simulink model "IPMSM_dq_Fault_R2020b_M"  (R2020b)
settings: Solver=VariableStepAuto  StartTime=0.0  StopTime=0.4  RelTol=1e-3
InitFcn:
  | clc
  | p=2;
  | R=3.45;
  | Ld=9.5e-3;
  | Lq=12e-3;
  | flux=0.55;
  | B=0;
  | J=0.0052;
  | 
  | L=(Ld+Lq)/2;
  | M=0.5e-3;
  | 
  | Rf=0.5;
  | 
  | TL=1e-6;
  | 
  | Ts=1e-6;
libraries: powerlib x6, powerlib_extras x3, simulink x1
settings Model: SimulationMode=accelerator  Creator=acer  LastModifiedBy=Beyond
settings DataIOCC: ReturnWorkspaceOutputs=off
settings DebuggingCC: ArithmeticOperatorsInVariantConditions=warning
settings SFSimCC: CustomCodeUndefinedFunction=UseInterfaceOnly
settings CodeAppCC: StateflowObjectComments=on

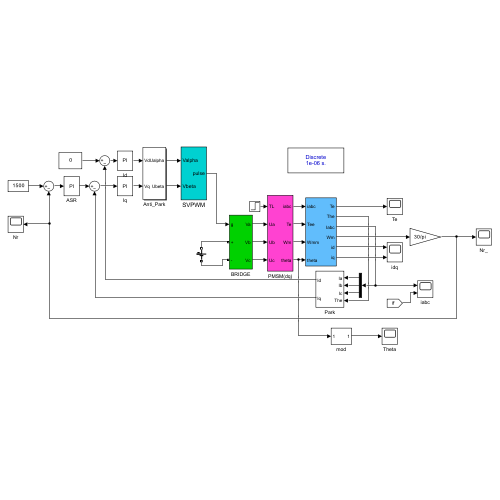
[thumbnail: Simulink's stored preview of the top-level diagram]
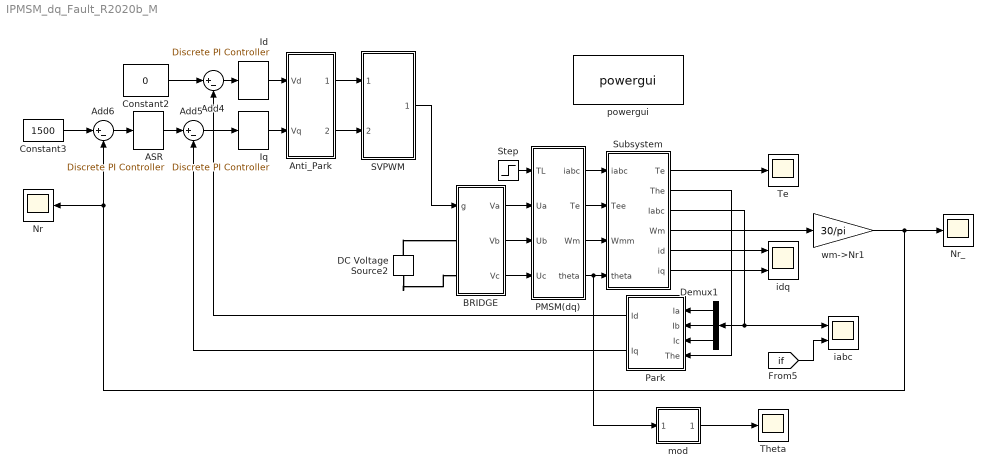
== system IPMSM_dq_Fault_R2020b_M ==
  ASR : powerlib_extras/Discrete  Control Blocks/Discrete PI Controller  Kp=0.15  Ki=10  Par_Limits=[30 -30]  Init=0  Ts=Ts
  Add4 : Sum  Inputs=|+-
  Add5 : Sum  Inputs=|+-
  Add6 : Sum  Inputs=|+-
  Anti_Park : Subsystem
  BRIDGE : Subsystem
  Constant2 : Constant  Value=0
  Constant3 : Constant  Value=1500
  DC Voltage Source2 : powerlib/Electrical Sources/DC Voltage Source  Amplitude=500  Measurements=None
  Demux1 : Demux  Outputs=3
  Id : powerlib_extras/Discrete  Control Blocks/Discrete PI Controller  Kp=Ld*5000  Ki=R*5000  Par_Limits=[500*0.9*sqrt(1/3) -500*0.9*sqrt(1/3)]  Init=0  Ts=Ts
  Iq : powerlib_extras/Discrete  Control Blocks/Discrete PI Controller  Kp=Lq*5000  Ki=R*5000  Par_Limits=[500*0.9*sqrt(1/3) -500*0.9*sqrt(1/3)]  Init=0  Ts=Ts
  Nr : Scope
  Nr_ : Scope
  PMSM(dq) : Subsystem
  Park : Subsystem
  SVPWM : Subsystem
  Step : Step  Time=0.1  Before=2  After=20  SampleTime=0
  Subsystem : Subsystem
  Te : Scope
  Theta : Scope
  iabc : Scope  NumInputPorts=2
  idq : Scope  NumInputPorts=2
  mod : Subsystem
  powergui : powerlib/powergui  SimulationMode=Discrete  SampleTime=1e-6  frequency=60  Iterations=50  frequencyindice=0  Pbase=100e6  ErrMax=1e-4  UnitsV=kV  UnitsW=MW  buscounter=0  FunctionMessages=off  echomessages=off  EnableUseOfTLC=off  CurrentSourceSwitches=off  DisableSnubberDevices=off  DisableRonSwitches=off  DisableVfSwitches=off  DisplayEquations=off  AutomaticDiscreteSolvers=off  SolverType=Tustin/Backward Euler (TBE)  Interpol=off  ExternalGateDelay=off  methode=off  Ts=100  x0status=blocks  SPID=off  SwTol=0  HookPort=off  NonlinearTolerance=1e-4  nMaxIteration=100  ContinueOnMaxIteration=off  RestoreLinks=warning  ResistiveCurrentMeasurement=off  Frange=[0:2:500]  Ylog=off  Xlog=on  ShowGrid=off  save=off  variable=ZData  structure=0  ZoomFFT=off  StartTime=0.0  cycles=1  DisplayStyle=1  fundamental=60  FreqAxis=off  MaxFrequency=1000  frequencyindicesteady=1  RmsSteady=1  display=off
  wm->Nr1 : Gain  Gain=30/pi
  wires:
  Id/1 -> Anti_Park/1(Vd)
  PMSM(dq)/3(Wm) -> Subsystem/3(Wmm)
  PMSM(dq)/2(Te) -> Subsystem/2(Tee)
  Park/1(Id) -> Add4/2
  Demux1/1 -> Park/1(Ia)
  PMSM(dq)/1(iabc) -> Subsystem/1(iabc)
  SVPWM/1(pulse) -> BRIDGE/1(g)
  Step/1 -> PMSM(dq)/1("TL ")
  Add5/1 -> Iq/1
  Anti_Park/2(Ubeta) -> SVPWM/2(Vbeta)
  Subsystem/2(The) -> Park/4(The)
  Subsystem/3(Iabc) -> iabc/1, Demux1/1
  Demux1/2 -> Park/2(Ib)
  Subsystem/6(iq) -> idq/2
  Subsystem/1(Te) -> Te/1
  Iq/1 -> Anti_Park/2(Vq)
  ASR/1 -> Add5/1
  Demux1/3 -> Park/3(Ic)
  Add4/1 -> Id/1
  Add6/1 -> ASR/1
  Subsystem/5(id) -> idq/1
  Anti_Park/1(Ualpha) -> SVPWM/1(Valpha)
  Constant2/1 -> Add4/1
  Constant3/1 -> Add6/1
  Park/2(Iq) -> Add5/2
  BRIDGE/1(Va) -> PMSM(dq)/2(Ua)
  BRIDGE/2(Vb) -> PMSM(dq)/3(Ub)
  BRIDGE/3(Vc) -> PMSM(dq)/4(Uc)
  wm->Nr1/1 -> Nr_/1, Nr/1, Add6/2
  mod/1(Out1) -> Theta/1
  PMSM(dq)/4(theta) -> mod/1(In1), Subsystem/4(theta)
  Subsystem/4(Wm) -> wm->Nr1/1
  [if] -> iabc/2
  connections:
  DC Voltage Source2/LConn1 -- BRIDGE/LConn2
  DC Voltage Source2/RConn1 -- BRIDGE/LConn1

== system IPMSM_dq_Fault_R2020b_M/Anti_Park ==
  Vd : Inport
  Vq : Inport  Port=2
  Fcn : Fcn  Expr=cos(u[3])*u[1]-sin(u[3])*u[2]
  Fcn1 : Fcn  Expr=sin(u[3])*u[1]+cos(u[3])*u[2]
  Mux1 : Mux  Inputs=3
  Ualpha : Outport
  Ubeta : Outport  Port=2
  wires:
  Fcn1/1 -> Ubeta/1
  Fcn/1 -> Ualpha/1
  Mux1/1 -> Fcn/1, Fcn1/1
  Vd/1 -> Mux1/1
  Vq/1 -> Mux1/2
  [Thedq] -> Mux1/3

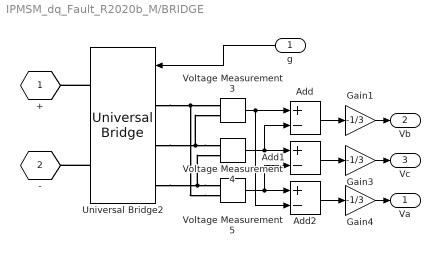
== system IPMSM_dq_Fault_R2020b_M/BRIDGE ==
  g : Inport
  Add : Sum  Inputs=+-
  Add1 : Sum  Inputs=+-
  Add2 : Sum  Inputs=+-
  Gain1 : Gain  Gain=-1/3
  Gain3 : Gain  Gain=-1/3
  Gain4 : Gain  Gain=-1/3
  Universal Bridge2 : powerlib/Power Electronics/Universal Bridge  Arms=3  SnubberResistance=1e5  SnubberCapacitance=inf  Device=IGBT / Diodes  Ron=1e-3  Lon=0  ForwardVoltages="[  0  0  ]"  ForwardVoltage=0  GTOparameters=[ 10e-6 , 20e-6 ]  IGBTparameters=[ 1e-6 , 2e-6 ]  Measurements=None  Measurements_2=None  converterType=Rectifier
  Voltage Measurement3 : powerlib/Measurements/Voltage Measurement  PhasorSimulation=off  OutputType=Complex  PSBequivalent=0
  Voltage Measurement4 : powerlib/Measurements/Voltage Measurement  PhasorSimulation=off  OutputType=Complex  PSBequivalent=0
  Voltage Measurement5 : powerlib/Measurements/Voltage Measurement  PhasorSimulation=off  OutputType=Complex  PSBequivalent=0
  + : PMIOPort  Tag=PMCPort  Side=Left
  - : PMIOPort  Tag=PMCPort  Port=2  Side=Left
  Va : Outport
  Vb : Outport  Port=2
  Vc : Outport  Port=3
  wires:
  g/1 -> Universal Bridge2/1
  Gain1/1 -> Vb/1
  Add2/1 -> Gain4/1
  Gain4/1 -> Va/1
  Voltage Measurement3/1 -> Add/1, Add2/2
  Voltage Measurement4/1 -> Add1/1, Add/2
  Add1/1 -> Gain3/1
  Voltage Measurement5/1 -> Add2/1, Add1/2
  Gain3/1 -> Vc/1
  Add/1 -> Gain1/1
  connections:
  Universal Bridge2/RConn1 -- +/RConn1
  Universal Bridge2/RConn2 -- -/RConn1
  Voltage Measurement5/LConn2 -- Universal Bridge2/LConn1 -- Voltage Measurement3/LConn1
  Voltage Measurement5/LConn1 -- Universal Bridge2/LConn3 -- Voltage Measurement4/LConn2
  Voltage Measurement4/LConn1 -- Universal Bridge2/LConn2 -- Voltage Measurement3/LConn2

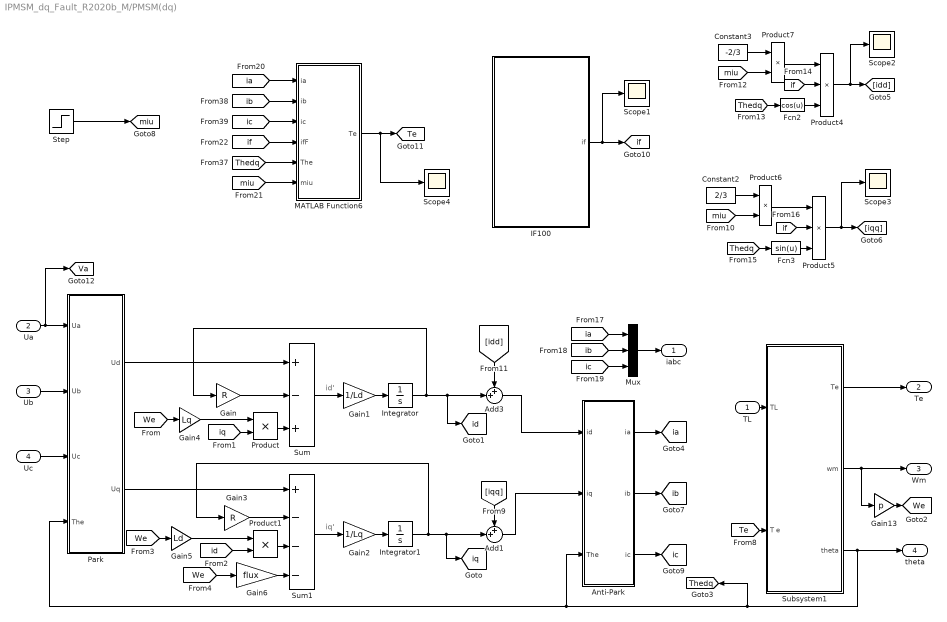
== system IPMSM_dq_Fault_R2020b_M/PMSM(dq) ==
  note: iq'
  note: id'
  "TL " : Inport
  Ua : Inport  Port=2
  Ub : Inport  Port=3
  Uc : Inport  Port=4
  Add1 : Sum  Inputs=++|
  Add3 : Sum  Inputs=++|
  Anti-Park : Subsystem
  Constant2 : Constant  Value=2/3
  Constant3 : Constant  Value=-2/3
  Fcn2 : Fcn  Expr=cos(u)
  Fcn3 : Fcn  Expr=sin(u)
  Gain : Gain  Gain=R
  Gain1 : Gain  Gain=1/Ld
  Gain13 : Gain  Gain=p
  Gain2 : Gain  Gain=1/Lq
  Gain3 : Gain  Gain=R
  Gain4 : Gain  Gain=Lq
  Gain5 : Gain  Gain=Ld
  Gain6 : Gain  Gain=flux
  IF100 : Subsystem
  Integrator : Integrator
  Integrator1 : Integrator
  MATLAB Function6 : MATLAB Function  TreatAsAtomicUnit=on
  Mux : Mux  Inputs=3
  Park : Subsystem
  Product{,1,6..7} (4 alike) : Product
  Product4 : Product  Inputs=3
  Product5 : Product  Inputs=3
  Scope{1..4} (4 alike) : Scope
  Step : Step  Time=0.2  After=0.12  SampleTime=0
  Subsystem1 : Subsystem
  Sum : Sum  Inputs=+-+
  Sum1 : Sum  Inputs=+---
  iabc : Outport
  Te : Outport  Port=2
  Wm : Outport  Port=3
  theta : Outport  Port=4
  tag scope: Te=global, Thedq=global, Va=global, We=global, ia=global, ib=global, ic=global, id=global, if=global, iq=global, miu=global
  wires:
  Ua/1 -> [Va], Park/1(Ua)
  Gain/1 -> Sum/2
  Sum/1 -> Gain1/1
  Subsystem1/1(Te) -> Te/1
  Gain4/1 -> Product/1
  Gain6/1 -> Sum1/4
  [id] -> Product1/2
  Ub/1 -> Park/2(Ub)
  Gain2/1 -> Integrator1/1
  [We] -> Gain6/1
  Subsystem1/3(theta) -> theta/1, [Thedq], Park/4(The), Anti-Park/3(The)
  Product1/1 -> Sum1/3
  [iq] -> Product/2
  Gain5/1 -> Product1/1
  Park/1(Ud) -> Sum/1
  Product/1 -> Sum/3
  Gain3/1 -> Sum1/2
  Gain1/1 -> Integrator/1
  Park/2(Uq) -> Sum1/1
  Subsystem1/2(wm) -> Gain13/1, Wm/1
  Sum1/1 -> Gain2/1
  Gain13/1 -> [We]
  [We] -> Gain4/1
  "TL "/1 -> Subsystem1/1(TL)
  [We] -> Gain5/1
  Uc/1 -> Park/3(Uc)
  Integrator/1 -> [id], Add3/2, Gain/1
  Integrator1/1 -> Gain3/1, [iq], Add1/2
  [idd] -> Add3/1
  [iqq] -> Add1/1
  Add3/1 -> Anti-Park/1(id)
  Add1/1 -> Anti-Park/2(iq)
  Product5/1 -> Scope3/1, [iqq]
  Product7/1 -> Product4/1
  [if] -> Product4/2
  Constant2/1 -> Product6/1
  [Thedq] -> Fcn3/1
  [miu] -> Product7/2
  Product6/1 -> Product5/1
  Fcn2/1 -> Product4/3
  Product4/1 -> Scope2/1, [idd]
  Constant3/1 -> Product7/1
  [Thedq] -> Fcn2/1
  [miu] -> Product6/2
  Fcn3/1 -> Product5/3
  [if] -> Product5/2
  Step/1 -> [miu]
  Anti-Park/1(ia) -> [ia]
  Anti-Park/2(ib) -> [ib]
  Anti-Park/3(ic) -> [ic]
  [Te] -> Subsystem1/2(T e)
  Mux/1 -> iabc/1
  [ia] -> Mux/1
  [ib] -> Mux/2
  [ic] -> Mux/3
  MATLAB Function6/1(Te) -> Scope4/1, [Te]
  [ia] -> MATLAB Function6/1(ia)
  [Thedq] -> MATLAB Function6/5(The)
  [ic] -> MATLAB Function6/3(ic)
  [ib] -> MATLAB Function6/2(ib)
  [if] -> MATLAB Function6/4(ifF)
  [miu] -> MATLAB Function6/6(miu)
  IF100/1(if) -> [if], Scope1/1

== system IPMSM_dq_Fault_R2020b_M/Park ==
  Ia : Inport
  Ib : Inport  Port=2
  Ic : Inport  Port=3
  The : Inport  Port=4
  Mux : Mux
  d : Fcn  Expr=(u(1)*cos(u(4))+u(2)*cos(u(4)-2/3*pi)+u(3)*cos(u(4)+2/3*pi))*2/3
  q : Fcn  Expr=-(u(1)*sin(u(4))+u(2)*sin(u(4)-2/3*pi)+u(3)*sin(u(4)+2/3*pi))*2/3
  Id : Outport
  Iq : Outport  Port=2
  wires:
  Mux/1 -> q/1, d/1
  Ia/1 -> Mux/1
  Ib/1 -> Mux/2
  d/1 -> Id/1
  The/1 -> Mux/4
  Ic/1 -> Mux/3
  q/1 -> Iq/1

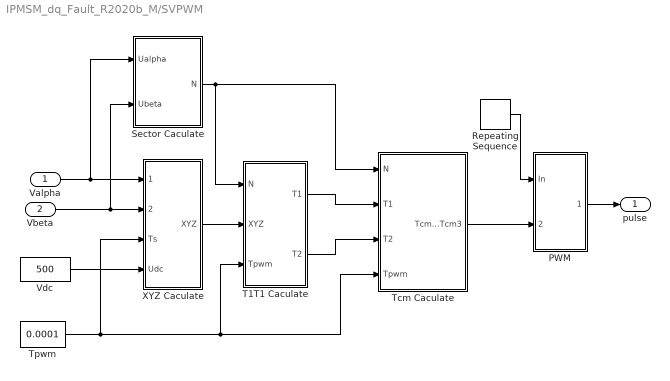
== system IPMSM_dq_Fault_R2020b_M/SVPWM ==
  Valpha : Inport
  Vbeta : Inport  Port=2
  PWM : Subsystem
  Repeating Sequence : simulink/Sources/Repeating Sequence  rep_seq_t=[0 0.00005 0.0001]  rep_seq_y=[0 0.00005 0]
  Sector Caculate : Subsystem
  T1T1 Caculate : Subsystem
  Tcm Caculate : Subsystem
  Tpwm : Constant  Value=0.0001
  Vdc : Constant  Value=500
  XYZ Caculate : Subsystem
  pulse : Outport
  wires:
  PWM/1(PWM) -> pulse/1
  Repeating Sequence/1 -> PWM/1(In)
  Vbeta/1 -> XYZ Caculate/2(Ubeta), Sector Caculate/2(Ubeta)
  T1T1 Caculate/1(T1) -> Tcm Caculate/2(T1)
  Valpha/1 -> XYZ Caculate/1(Ualpha), Sector Caculate/1(Ualpha)
  T1T1 Caculate/2(T2) -> Tcm Caculate/3(T2)
  Sector Caculate/1("N ") -> Tcm Caculate/1(N), T1T1 Caculate/1(N)
  XYZ Caculate/1(XYZ) -> T1T1 Caculate/2(XYZ)
  Tpwm/1 -> XYZ Caculate/3(Ts), Tcm Caculate/4(Tpwm), T1T1 Caculate/3(Tpwm)
  Vdc/1 -> XYZ Caculate/4(Udc)
  Tcm Caculate/1(Tcm1 Tcm2 Tcm3) -> PWM/2(Tcm123)

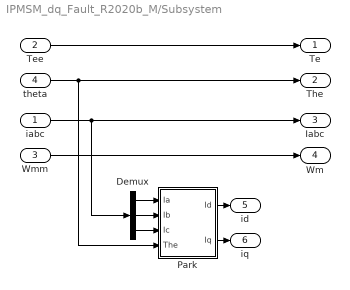
== system IPMSM_dq_Fault_R2020b_M/Subsystem ==
  iabc : Inport
  Tee : Inport  Port=2
  Wmm : Inport  Port=3
  theta : Inport  Port=4
  Demux : Demux  Outputs=3
  Park : Subsystem
  Te : Outport
  The : Outport  Port=2
  Iabc : Outport  Port=3
  Wm : Outport  Port=4
  id : Outport  Port=5
  iq : Outport  Port=6
  wires:
  iabc/1 -> Demux/1, Iabc/1
  Tee/1 -> Te/1
  theta/1 -> Park/4(The), The/1
  Wmm/1 -> Wm/1
  Demux/1 -> Park/1(Ia)
  Demux/2 -> Park/2(Ib)
  Demux/3 -> Park/3(Ic)
  Park/1(Id) -> id/1
  Park/2(Iq) -> iq/1

== system IPMSM_dq_Fault_R2020b_M/mod ==
  In1 : Inport
  Constant : Constant  Value=2*pi
  Math Function : Math  Operator=mod  SignedPower=on  SaturateOnIntegerOverflow=on
  Out1 : Outport
  wires:
  Constant/1 -> Math Function/2
  In1/1 -> Math Function/1
  Math Function/1 -> Out1/1

== system IPMSM_dq_Fault_R2020b_M/PMSM(dq)/Anti-Park ==
  id : Inport
  iq : Inport  Port=2
  The : Inport  Port=3
  Mux : Mux  Inputs=3
  a : Fcn  Expr=u(1)*cos(u(3))-u(2)*sin(u(3))
  b : Fcn  Expr=u(1)*cos(u(3)-2/3*pi)-u(2)*sin(u(3)-2/3*pi)
  c : Fcn  Expr=u(1)*cos(u(3)+2/3*pi)-u(2)*sin(u(3)+2/3*pi)
  ia : Outport
  ib : Outport  Port=2
  ic : Outport  Port=3
  wires:
  b/1 -> ib/1
  The/1 -> Mux/3
  a/1 -> ia/1
  id/1 -> Mux/1
  iq/1 -> Mux/2
  Mux/1 -> c/1, a/1, b/1
  c/1 -> ic/1

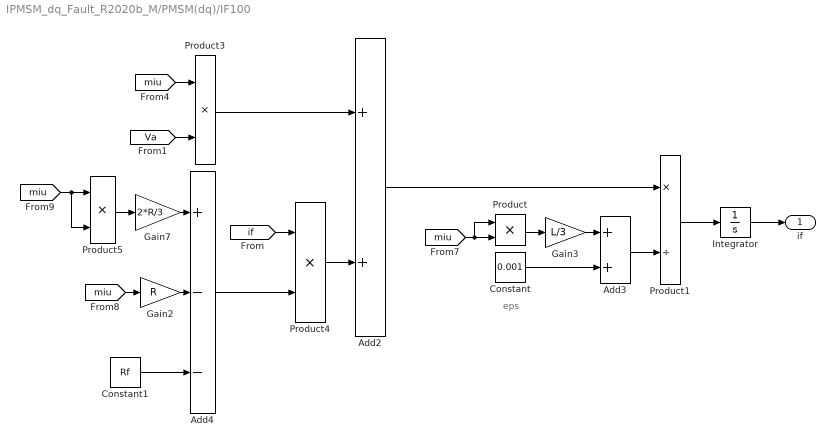
== system IPMSM_dq_Fault_R2020b_M/PMSM(dq)/IF100 ==
  note: eps
  Add2 : Sum
  Add3 : Sum
  Add4 : Sum  Inputs=+--
  Constant : Constant  Value=0.001
  Constant1 : Constant  Value=Rf
  Gain2 : Gain  Gain=R
  Gain3 : Gain  Gain=L/3
  Gain7 : Gain  Gain=2*R/3
  Integrator : Integrator  InitialCondition=0.2
  Product{,3..5} (4 alike) : Product
  Product1 : Product  Inputs=*/
  if : Outport
  wires:
  [Va] -> Product3/2
  [miu] -> Product3/1
  Product3/1 -> Add2/1
  [miu] -> Product/2, Product/1
  Product/1 -> Gain3/1
  Add2/1 -> Product1/1
  Gain3/1 -> Add3/1
  Add3/1 -> Product1/2
  Constant/1 -> Add3/2
  Integrator/1 -> if/1
  Product1/1 -> Integrator/1
  Add4/1 -> Product4/2
  [if] -> Product4/1
  Product4/1 -> Add2/2
  Constant1/1 -> Add4/3
  [miu] -> Gain2/1
  Gain2/1 -> Add4/2
  Gain7/1 -> Add4/1
  Product5/1 -> Gain7/1
  [miu] -> Product5/2, Product5/1

== system IPMSM_dq_Fault_R2020b_M/PMSM(dq)/Park ==
  Ua : Inport
  Ub : Inport  Port=2
  Uc : Inport  Port=3
  The : Inport  Port=4
  Mux : Mux
  d : Fcn  Expr=(u(1)*cos(u(4))+u(2)*cos(u(4)-2/3*pi)+u(3)*cos(u(4)+2/3*pi))*2/3
  q : Fcn  Expr=-(u(1)*sin(u(4))+u(2)*sin(u(4)-2/3*pi)+u(3)*sin(u(4)+2/3*pi))*2/3
  Ud : Outport
  Uq : Outport  Port=2
  wires:
  Mux/1 -> q/1, d/1
  Ua/1 -> Mux/1
  Ub/1 -> Mux/2
  d/1 -> Ud/1
  The/1 -> Mux/4
  Uc/1 -> Mux/3
  q/1 -> Uq/1

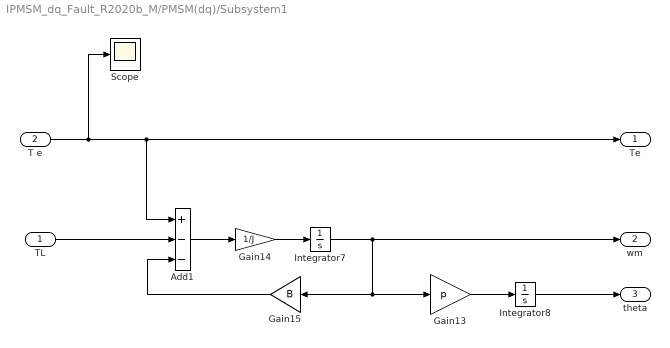
== system IPMSM_dq_Fault_R2020b_M/PMSM(dq)/Subsystem1 ==
  TL : Inport
  T e : Inport  Port=2
  Add1 : Sum  Inputs=+--
  Gain13 : Gain  Gain=p
  Gain14 : Gain  Gain=1/J
  Gain15 : Gain  Gain=B
  Integrator7 : Integrator
  Integrator8 : Integrator
  Scope : Scope
  Te : Outport
  wm : Outport  Port=2
  theta : Outport  Port=3
  wires:
  TL/1 -> Add1/2
  Add1/1 -> Gain14/1
  T e/1 -> Scope/1, Te/1, Add1/1
  Gain14/1 -> Integrator7/1
  Gain15/1 -> Add1/3
  Gain13/1 -> Integrator8/1
  Integrator8/1 -> theta/1
  Integrator7/1 -> wm/1, Gain13/1, Gain15/1

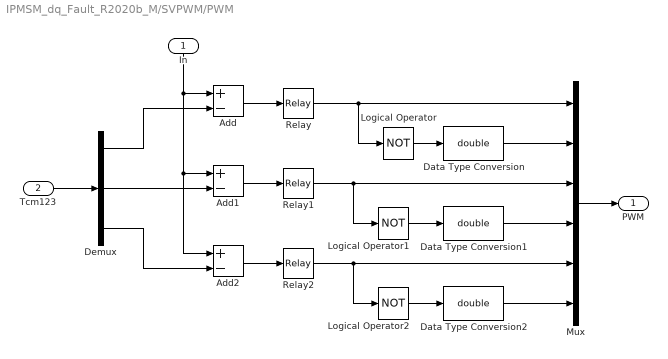
== system IPMSM_dq_Fault_R2020b_M/SVPWM/PWM ==
  In : Inport
  Tcm123 : Inport  Port=2
  Add : Sum  Inputs=+-
  Add1 : Sum  Inputs=+-
  Add2 : Sum  Inputs=+-
  Data Type Conversion : DataTypeConversion  OutDataTypeStr=double
  Data Type Conversion1 : DataTypeConversion  OutDataTypeStr=double
  Data Type Conversion2 : DataTypeConversion  OutDataTypeStr=double
  Demux : Demux  Outputs=3
  Logical Operator : Logic  Operator=NOT  AllPortsSameDT=off  OutDataTypeStr=boolean
  Logical Operator1 : Logic  Operator=NOT  AllPortsSameDT=off  OutDataTypeStr=boolean
  Logical Operator2 : Logic  Operator=NOT  AllPortsSameDT=off  OutDataTypeStr=boolean
  Mux : Mux  Inputs=6
  Relay : Relay  OffSwitchValue=-eps
  Relay1 : Relay  OffSwitchValue=-eps
  Relay2 : Relay  OffSwitchValue=-eps
  PWM : Outport
  wires:
  Demux/3 -> Add2/2
  Demux/2 -> Add1/2
  Demux/1 -> Add/2
  Relay2/1 -> Mux/5, Logical Operator2/1
  Relay1/1 -> Mux/3, Logical Operator1/1
  Relay/1 -> Logical Operator/1, Mux/1
  Mux/1 -> PWM/1
  Data Type Conversion/1 -> Mux/2
  Data Type Conversion1/1 -> Mux/4
  Data Type Conversion2/1 -> Mux/6
  Logical Operator2/1 -> Data Type Conversion2/1
  Logical Operator1/1 -> Data Type Conversion1/1
  Logical Operator/1 -> Data Type Conversion/1
  Add1/1 -> Relay1/1
  Add2/1 -> Relay2/1
  Add/1 -> Relay/1
  In/1 -> Add/1, Add2/1, Add1/1
  Tcm123/1 -> Demux/1

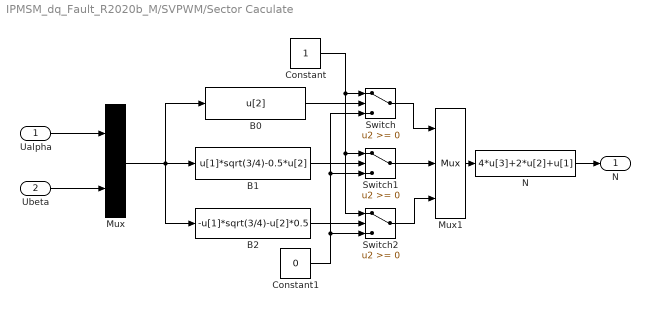
== system IPMSM_dq_Fault_R2020b_M/SVPWM/Sector Caculate ==
  Ualpha : Inport
  Ubeta : Inport  Port=2
  B0 : Fcn  Expr=u[2]
  B1 : Fcn  Expr=u[1]*sqrt(3/4)-0.5*u[2]
  B2 : Fcn  Expr=-u[1]*sqrt(3/4)-u[2]*0.5
  Constant : Constant
  Constant1 : Constant  Value=0
  Mux : Mux  Inputs=2
  Mux1 : Mux  Inputs=3
  N : Fcn  Expr=4*u[3]+2*u[2]+u[1]
  Switch : Switch
  Switch1 : Switch
  Switch2 : Switch
  "N " : Outport
  wires:
  Switch2/1 -> Mux1/3
  Switch/1 -> Mux1/1
  Ualpha/1 -> Mux/1
  Ubeta/1 -> Mux/2
  Mux/1 -> B2/1, B1/1, B0/1
  B0/1 -> Switch/2
  B1/1 -> Switch1/2
  B2/1 -> Switch2/2
  Constant/1 -> Switch/1, Switch2/1, Switch1/1
  Constant1/1 -> Switch/3, Switch1/3, Switch2/3
  Switch1/1 -> Mux1/2
  Mux1/1 -> N/1
  N/1 -> "N "/1

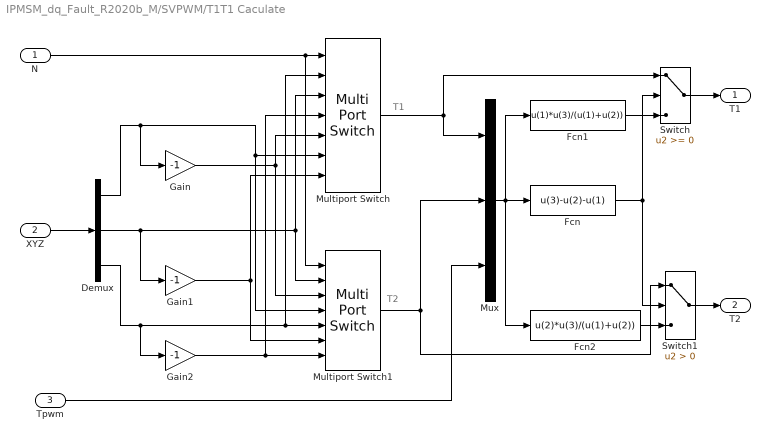
== system IPMSM_dq_Fault_R2020b_M/SVPWM/T1T1 Caculate ==
  note: T1
  note: T2
  N : Inport
  XYZ : Inport  Port=2
  Tpwm : Inport  Port=3
  Demux : Demux  Outputs=3
  Fcn : Fcn  Expr=u(3)-u(2)-u(1)
  Fcn1 : Fcn  Expr=u(1)*u(3)/(u(1)+u(2))
  Fcn2 : Fcn  Expr=u(2)*u(3)/(u(1)+u(2))
  Gain : Gain  Gain=-1
  Gain1 : Gain  Gain=-1
  Gain2 : Gain  Gain=-1
  Multiport Switch : MultiPortSwitch  Inputs=6
  Multiport Switch1 : MultiPortSwitch  Inputs=6
  Mux : Mux  Inputs=3
  Switch : Switch
  Switch1 : Switch  Criteria=u2 > Threshold
  T1 : Outport
  T2 : Outport  Port=2
  wires:
  Tpwm/1 -> Mux/3
  XYZ/1 -> Demux/1
  Switch1/1 -> T2/1
  Switch/1 -> T1/1
  Fcn2/1 -> Switch1/3
  Fcn1/1 -> Switch/3
  Fcn/1 -> Switch/2, Switch1/2
  Mux/1 -> Fcn1/1, Fcn/1, Fcn2/1
  Multiport Switch/1 -> Switch/1, Mux/1
  Multiport Switch1/1 -> Switch1/1, Mux/2
  N/1 -> Multiport Switch/1, Multiport Switch1/1
  Demux/2 -> Multiport Switch/3, Multiport Switch1/2, Gain1/1
  Demux/3 -> Multiport Switch1/5, Multiport Switch/2, Gain2/1
  Demux/1 -> Multiport Switch/6, Multiport Switch1/4, Gain/1
  Gain/1 -> Multiport Switch1/3, Multiport Switch/5
  Gain2/1 -> Multiport Switch/4, Multiport Switch1/7
  Gain1/1 -> Multiport Switch1/6, Multiport Switch/7

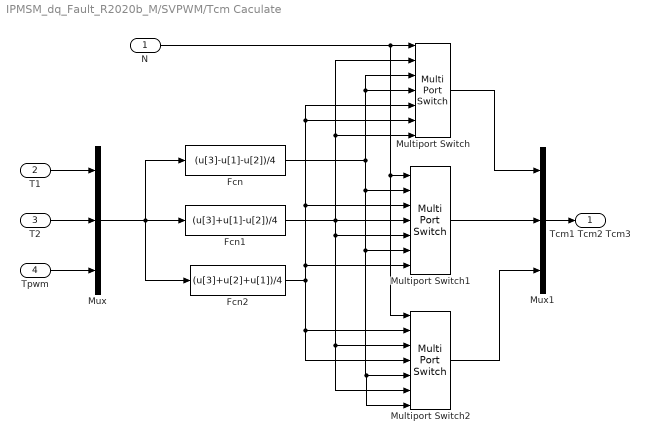
== system IPMSM_dq_Fault_R2020b_M/SVPWM/Tcm Caculate ==
  N : Inport
  T1 : Inport  Port=2
  T2 : Inport  Port=3
  Tpwm : Inport  Port=4
  Fcn : Fcn  Expr=(u[3]-u[1]-u[2])/4
  Fcn1 : Fcn  Expr=(u[3]+u[1]-u[2])/4
  Fcn2 : Fcn  Expr=(u[3]+u[2]+u[1])/4
  Multiport Switch : MultiPortSwitch  Inputs=6
  Multiport Switch1 : MultiPortSwitch  Inputs=6
  Multiport Switch2 : MultiPortSwitch  Inputs=6
  Mux : Mux  Inputs=3
  Mux1 : Mux  Inputs=3
  Tcm1 Tcm2 Tcm3 : Outport
  wires:
  Mux/1 -> Fcn2/1, Fcn/1, Fcn1/1
  Tpwm/1 -> Mux/3
  T2/1 -> Mux/2
  T1/1 -> Mux/1
  Multiport Switch2/1 -> Mux1/3
  Multiport Switch1/1 -> Mux1/2
  Multiport Switch/1 -> Mux1/1
  Mux1/1 -> Tcm1 Tcm2 Tcm3/1
  Fcn/1 -> Multiport Switch/3, Multiport Switch/4, Multiport Switch1/6, Multiport Switch2/5, Multiport Switch2/7, Multiport Switch1/2
  Fcn1/1 -> Multiport Switch1/5, Multiport Switch2/3, Multiport Switch2/6, Multiport Switch1/4, Multiport Switch/7, Multiport Switch/2
  Fcn2/1 -> Multiport Switch/5, Multiport Switch/6, Multiport Switch1/3, Multiport Switch1/7, Multiport Switch2/2, Multiport Switch2/4
  N/1 -> Multiport Switch2/1, Multiport Switch1/1, Multiport Switch/1

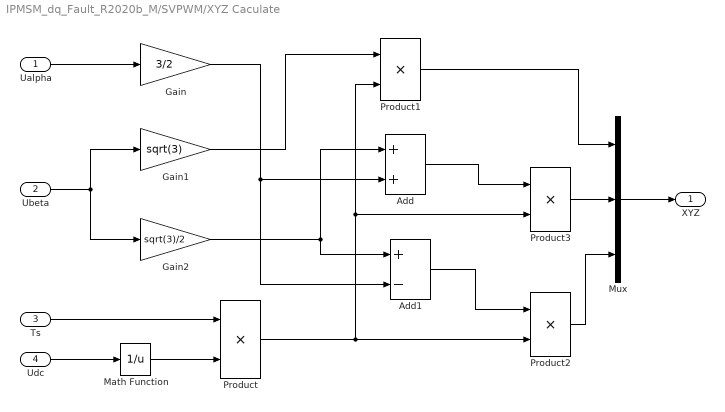
== system IPMSM_dq_Fault_R2020b_M/SVPWM/XYZ Caculate ==
  Ualpha : Inport
  Ubeta : Inport  Port=2
  Ts : Inport  Port=3
  Udc : Inport  Port=4
  Add : Sum
  Add1 : Sum  Inputs=+-
  Gain : Gain  Gain=3/2
  Gain1 : Gain  Gain=sqrt(3)
  Gain2 : Gain  Gain=sqrt(3)/2
  Math Function : Math  Operator=reciprocal  SignedPower=on  SaturateOnIntegerOverflow=on
  Mux : Mux  Inputs=3
  Product{,1..3} (4 alike) : Product  RndMeth=Zero
  XYZ : Outport
  wires:
  Mux/1 -> XYZ/1
  Product1/1 -> Mux/1
  Product3/1 -> Mux/2
  Product2/1 -> Mux/3
  Ualpha/1 -> Gain/1
  Ubeta/1 -> Gain2/1, Gain1/1
  Udc/1 -> Math Function/1
  Math Function/1 -> Product/2
  Ts/1 -> Product/1
  Gain1/1 -> Product1/1
  Product/1 -> Product2/2, Product1/2, Product3/2
  Gain/1 -> Add1/2, Add/2
  Gain2/1 -> Add/1, Add1/1
  Add1/1 -> Product2/1
  Add/1 -> Product3/1

== system IPMSM_dq_Fault_R2020b_M/Subsystem/Park ==
  Ia : Inport
  Ib : Inport  Port=2
  Ic : Inport  Port=3
  The : Inport  Port=4
  Mux : Mux
  d : Fcn  Expr=(u(1)*cos(u(4))+u(2)*cos(u(4)-2/3*pi)+u(3)*cos(u(4)+2/3*pi))*2/3
  q : Fcn  Expr=-(u(1)*sin(u(4))+u(2)*sin(u(4)-2/3*pi)+u(3)*sin(u(4)+2/3*pi))*2/3
  Id : Outport
  Iq : Outport  Port=2
  wires:
  Mux/1 -> q/1, d/1
  Ia/1 -> Mux/1
  Ib/1 -> Mux/2
  d/1 -> Id/1
  The/1 -> Mux/4
  Ic/1 -> Mux/3
  q/1 -> Iq/1

== matlab function IPMSM_dq_Fault_R2020b_M/PMSM(dq)/MATLAB Function6 ==
  data: ia input; ib input; ic input; ifF input; The input; miu input; Te output
function Te = fcn(ia,ib,ic,ifF,The,miu)
%参数设置
p = 2;
flux=0.55;

ga = (1-miu)*ia*sin(The);
%上面(1-miu)留？舍？
gb = ib*sin(The-2/3*pi);
gc = ic*sin(The+2/3*pi);

gf = miu*ifF*sin(The);
%电磁转矩

Te =-1*p*flux*(ga+gb+gc-gf);
end
